simulink model "constant_speed_platoon"  (R2017b)
settings: Solver=VariableStepAuto  StartTime=0.0  StopTime=10.0  RelTol=1e-3
values from neighbouring files (symbols this model uses):
  A_C = [0,0,0,0,0,0,0,0,0,0 ... (first row only)    [param.m]
  D_C = [v ... (first row only)    [param.m]
  K1 = 1    [param.m]
  start = [0;1.5;0;-1.5;-3;3;-3;0;-3;-3]    [param.m]
settings Model: Creator=yunfei  LastModifiedBy=yunfei

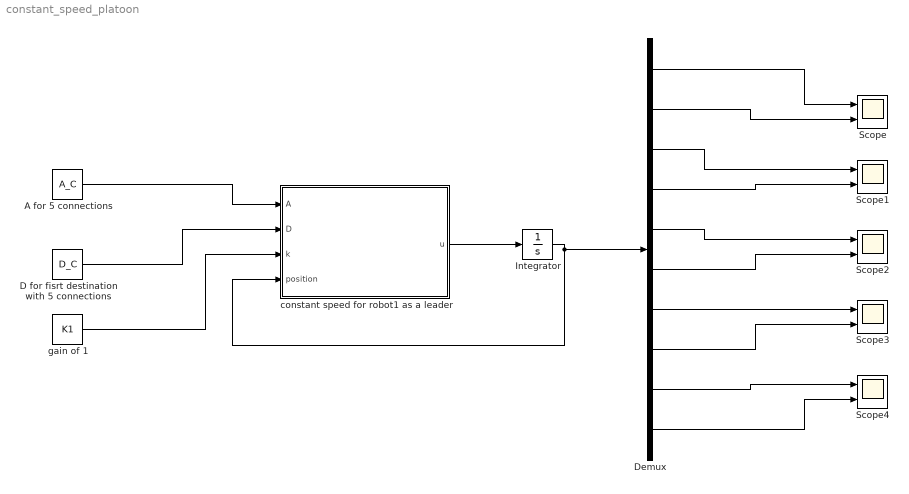
== system constant_speed_platoon ==
  A for 5 connections : Constant  Value=A_C
  "D for fisrt destination with 5 connections " : Constant  Value=D_C
  Demux : Demux  Outputs=10
  Integrator : Integrator  InitialCondition=start
  Scope{,1..4} (5 alike) : Scope  NumInputPorts=2
  constant speed for robot1 as a leader : MATLAB Function  TreatAsAtomicUnit=on
  gain of 1 : Constant  Value=K1
  wires:
  Demux/6 -> Scope2/2
  Demux/10 -> Scope4/2
  Demux/5 -> Scope2/1
  Demux/8 -> Scope3/2
  Integrator/1 -> constant speed for robot1 as a leader/4(position), Demux/1
  Demux/4 -> Scope1/2
  constant speed for robot1 as a leader/1(u) -> Integrator/1
  Demux/7 -> Scope3/1
  Demux/9 -> Scope4/1
  "D for fisrt destination with 5 connections "/1 -> constant speed for robot1 as a leader/2(D)
  Demux/1 -> Scope/1
  A for 5 connections/1 -> constant speed for robot1 as a leader/1(A)
  Demux/2 -> Scope/2
  Demux/3 -> Scope1/1
  gain of 1/1 -> constant speed for robot1 as a leader/3(k)

== matlab function constant_speed_platoon/constant speed for robot1 as a leader ==
  data: A input; u output; D input; k input; position input
function u = fcn(A, D, k, position)
    u = k.*A * position + D;
end
